simulink model "model2"  (R2015a)
settings: Solver=ode45  StartTime=0.0  StopTime=50  FixedStep=400  RelTol=1e-3
values from neighbouring files (symbols this model uses):
  g = 9.81    [balancin.m]
  Id = (1/2)*md*(Re^2+Ri^2)    (= 0.000284581170525)    [balancin.m]
  Is = ms*(l^2)    (= 0.0014779559807)    [balancin.m]
  K = [0 0 0]    [balancin.m]
  Kfric = 1.5    [balancin.m]
  l = 0.12    [balancin.m]
  ms = 1.1*md    (= 0.102635831993)    [balancin.m]
settings Model: Creator=Richa  LastModifiedBy=Richa

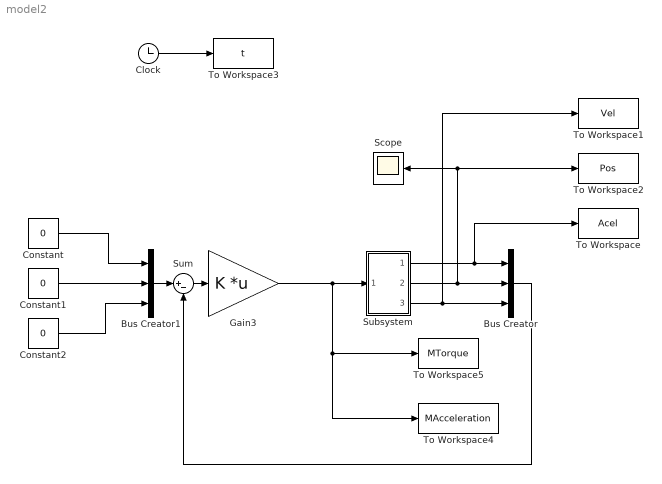
== system model2 ==
  Bus Creator : BusCreator  Inputs=3
  Bus Creator1 : BusCreator  Inputs=3
  Clock : Clock
  Constant : Constant  Value=0
  Constant1 : Constant  Value=0
  Constant2 : Constant  Value=0
  Gain3 : Gain  Gain=K  Multiplication=Matrix(K*u) (u vector)
  Scope : Scope
  Subsystem : Subsystem
  Sum : Sum  Inputs=|+-
  To Workspace : ToWorkspace  VariableName=Acel  SampleTime=-1
  To Workspace1 : ToWorkspace  VariableName=Vel  SampleTime=-1
  To Workspace2 : ToWorkspace  VariableName=Pos  SampleTime=-1
  To Workspace3 : ToWorkspace  VariableName=t  SampleTime=-1
  To Workspace4 : ToWorkspace  VariableName=MAcceleration  SampleTime=-1
  To Workspace5 : ToWorkspace  VariableName=MTorque  SampleTime=-1
  wires:
  Clock/1 -> To Workspace3/1
  Bus Creator1/1 -> Sum/1
  Bus Creator/1 -> Sum/2
  Sum/1 -> Gain3/1
  Constant/1 -> Bus Creator1/1
  Constant1/1 -> Bus Creator1/2
  Constant2/1 -> Bus Creator1/3
  Subsystem/3(Out3) -> Bus Creator/3, To Workspace1/1
  Subsystem/2(Out2) -> Bus Creator/2, To Workspace2/1, Scope/1
  Subsystem/1(Out1) -> Bus Creator/1, To Workspace/1
  Gain3/1 -> To Workspace4/1, To Workspace5/1, Subsystem/1(In1)

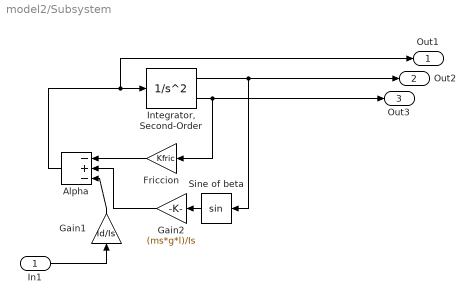
== system model2/Subsystem ==
  In1 : Inport
  Alpha : Sum  Inputs=-+-
  Friccion : Gain  Gain=Kfric
  Gain1 : Gain  Gain=Id/Is
  Gain2 : Gain  Gain=(ms*g*l)/Is
  "Integrator, Second-Order" : SecondOrderIntegrator  ICX=0.01  UpperLimitX=(5/16)*pi  LowerLimitX=-(5/16)*pi  ICDXDT=0
  Sine of beta : Trigonometry
  Out1 : Outport
  Out2 : Outport  Port=2
  Out3 : Outport  Port=3
  wires:
  In1/1 -> Gain1/1
  Sine of beta/1 -> Gain2/1
  Alpha/1 -> Out1/1, "Integrator, Second-Order"/1
  "Integrator, Second-Order"/1 -> Out2/1, Sine of beta/1
  Gain1/1 -> Alpha/3
  Friccion/1 -> Alpha/1
  Gain2/1 -> Alpha/2
  "Integrator, Second-Order"/2 -> Friccion/1, Out3/1
